simulink model "ACT_Lab4_dee"  (R2018b)
settings: Solver=ode45  StartTime=0.0  StopTime=100  RelTol=1e-3  AbsTol=1e-6
settings Model: ExtModeTrigMode=oneshot  ExtModeArmWhenConnect=off  Creator=sanjai  LastModifiedBy=gaura
settings DataIOCC: SaveFormat=Array  SignalLoggingSaveFormat=ModelDataLogs  SaveOutput=off  SaveTime=off
settings OptimizationCC: BlockReduction=off  BooleanDataType=off
settings DebuggingCC: SaveWithParameterizedLinksMsg=none  UnderspecifiedInitializationDetection=Classic  MergeDetectMultiDrivingBlocksExec=none  SignalResolutionControl=TryResolveAllWithWarning  MultiTaskDSMMsg=warning  MultiTaskCondExecSysMsg=none
settings HardwareCC: TargetUnknown=on
settings ModelReferenceCC: PropagateSignalLabelsOutOfModel=off
settings GRTTargetCC: CombineOutputUpdateFcns=off  GRTInterface=on

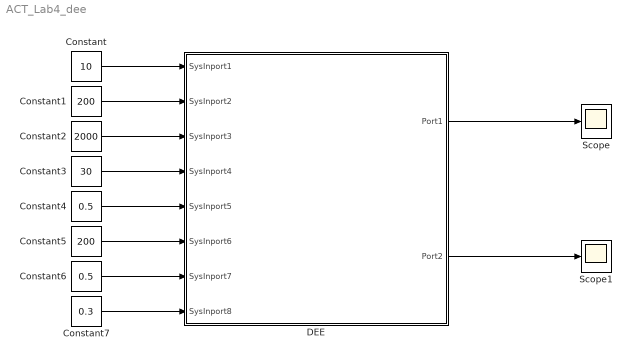
== system ACT_Lab4_dee ==
  Constant : Constant  Value=10
  Constant1 : Constant  Value=200
  Constant2 : Constant  Value=2000
  Constant3 : Constant  Value=30
  Constant4 : Constant  Value=0.5
  Constant5 : Constant  Value=200
  Constant6 : Constant  Value=0.5
  Constant7 : Constant  Value=0.3
  DEE : Subsystem  mask(Differential Equation Editor (DEE)){}
      settings: OpenFcn=diffeqed
      mask Display: disp('Differential Equation\n Editor')
  Scope : Scope
  Scope1 : Scope
  wires:
  Constant/1 -> DEE/1(SysInport1)
  Constant1/1 -> DEE/2(SysInport2)
  Constant2/1 -> DEE/3(SysInport3)
  Constant3/1 -> DEE/4(SysInport4)
  Constant4/1 -> DEE/5(SysInport5)
  Constant5/1 -> DEE/6(SysInport6)
  Constant6/1 -> DEE/7(SysInport7)
  Constant7/1 -> DEE/8(SysInport8)
  DEE/1(Port1) -> Scope/1
  DEE/2(Port2) -> Scope1/1

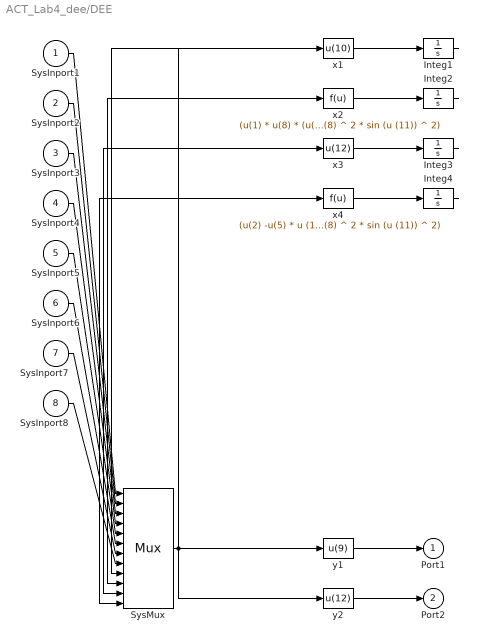
== system ACT_Lab4_dee/DEE ==
  SysInport1 : Inport
  SysInport2 : Inport  Port=2
  SysInport3 : Inport  Port=3
  SysInport4 : Inport  Port=4
  SysInport5 : Inport  Port=5
  SysInport6 : Inport  Port=6
  SysInport7 : Inport  Port=7
  SysInport8 : Inport  Port=8
  Integ{1..4} (4 alike) : Integrator  InitialCondition=1
  SysMux : Mux  Inputs=12
  x1 : Fcn  Expr=u(10)
  x2 : Fcn  Expr=(u(1) * u(8) * (u(2) -u(5) * u (12)) * sin (u (11))) / (u(7) * u(6) - u(1) ^ 2 * u(8) ^ 2 * sin (u (11)) ^ 2) + (u(7) * u(1) * u(8) * u (12) ^ 2 * cos (u (11))) / (u(7) * u(6) - u(1) ^ 2 * u(8) ^ 2 * sin (u (11)) ^ 2) -u(7) * u(3) * u (9) / (u(7) * u(6 ) - u(1) ^ 2 * u(8) ^ 2 * sin (u (11)) ^ 2) -u(7) * u(4) * u (10) / (u(7) * u(6 ) - u(1) ^ 2 * u(8) ^ 2 * sin (u (11)) ^ 2)
  x3 : Fcn  Expr=u(12)
  x4 : Fcn  Expr=(u(2) -u(5) * u (12)) / u(7) + (u(1) ^ 2 * u(8) ^ 2 * (u(2) - u(5) * u (12)) * sin (u (11)) ^ 2) / (u(7) * (u(7) * u(6) - u(1) ^ 2 * u(8 ) ^ 2 * sin (u (11)) ^ 2)) + u(1) ^ 2 * u(8) ^ 2 * u (12) ^ 2 * cos (u (11)) * sin (u (11)) / (u(7) * u(6) -u(1) ^ 2 * u(8) ^ 2 * sin (u (11)) ^ 2) -u(1) * u(8) * u(3 ) * u (9) * sin (u (11)) / (u(7) * u(6) -u(1) ^ 2 * u(8) ^ 2 * sin (u (11)) ^ 2) -u(1) * u(8) * u(4) * u (10) * sin (u (11)) / (u(7) * u(6) -u(1) ^ 2 * u(8) ^ 2 * sin (u (11)) ^ 2)
  y1 : Fcn  Expr=u(9)
  y2 : Fcn  Expr=u(12)
  Port1 : Outport
  Port2 : Outport  Port=2
  wires:
  SysInport1/1 -> SysMux/1
  SysInport2/1 -> SysMux/2
  SysInport3/1 -> SysMux/3
  SysInport4/1 -> SysMux/4
  SysInport5/1 -> SysMux/5
  SysInport6/1 -> SysMux/6
  SysInport7/1 -> SysMux/7
  SysInport8/1 -> SysMux/8
  SysMux/1 -> x1/1, x2/1, x3/1, x4/1, y1/1, y2/1
  x1/1 -> Integ1/1
  Integ1/1 -> SysMux/9
  x2/1 -> Integ2/1
  Integ2/1 -> SysMux/10
  x3/1 -> Integ3/1
  Integ3/1 -> SysMux/11
  x4/1 -> Integ4/1
  Integ4/1 -> SysMux/12
  y1/1 -> Port1/1
  y2/1 -> Port2/1
